simulink model "AeroPistonEngineSimulator"  (R2026a)
settings: Solver=VariableStepAuto  StopTime=1000
model workspace (MAT data in the model file):
  linear_friction_constant = 0.001
values from neighbouring files (symbols this model uses):
  C_oil = 2500    [engine_params.m]
  CHT_capacity = 100    [engine_params.m]
  drift_ialt = 0    [engine_params.m]
  drift_injd = 0    [engine_params.m]
  drift_injt = 0    [engine_params.m]
  drift_vbatt = 0    [engine_params.m]
  EGT_tau = 0.8    [engine_params.m]
  fault_ramp_time = 300    [engine_params.m]
  friction_a = 0.001    [engine_params.m]
  friction_b = 0.00005    (= 5e-05)    [engine_params.m]
  J_engine = 0.05    [engine_params.m]
  k_c = 5    [engine_params.m]
  k_h = 100    [engine_params.m]
  k_oil_cool = 0.05    [engine_params.m]
  k_oil_heat = 8    [engine_params.m]
  k_oil_pressure_rpm = 0.015    [engine_params.m]
  k_oil_pressure_temp = 0.000075    (= 7.5e-05)    [engine_params.m]
  RPM_max = 7500    [engine_params.m]
  sat_ialt = [0 40]    [engine_params.m]
  sat_injd = [0 30]    [engine_params.m]
  sat_injt = [0 60]    [engine_params.m]
  sat_vbatt = [0 36]    [engine_params.m]
  T_max = 10    [engine_params.m]
  tau_ialt_sensor = 0.1    [engine_params.m]
  tau_injd_sensor = 0.05    [engine_params.m]
  tau_injt_sensor = 0.05    [engine_params.m]
  tau_vbatt_sensor = 0.1    [engine_params.m]
  Ts_telemetry_slow = 0.5    [engine_params.m]
  Ts_telemetry_std = 0.1    [engine_params.m]
undefined symbols (not defined in the file or in its folder): DiscIntNeverNeededParam, elec, inj
libraries: simulink x27
settings Model: Creator=ambar  LastModifiedBy=vedanth
settings DataIOCC: LoadExternalInput=on

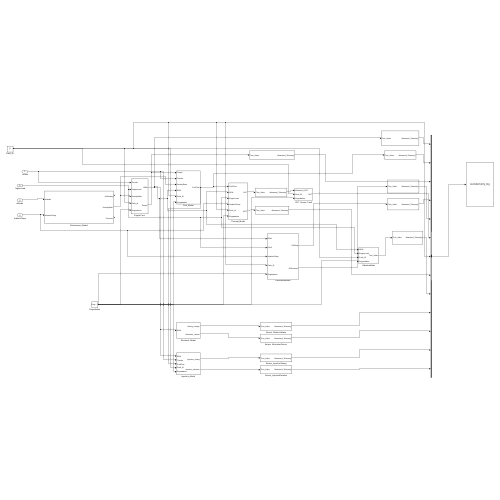
[thumbnail: Simulink's stored preview of the top-level diagram]
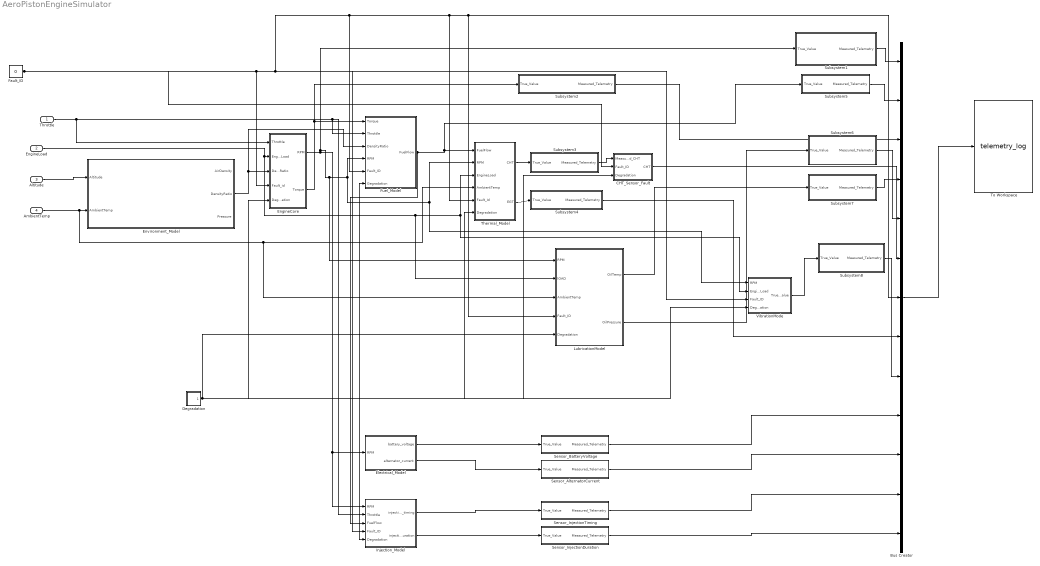
== system AeroPistonEngineSimulator ==
  Throttle : Inport
  EngineLoad : Inport  Port=2
  Altitude : Inport  Port=3
  AmbientTemp : Inport  Port=4
  Bus Creator : BusCreator  Inputs=13
  CHT_Sensor_Fault : Subsystem  Description=Fault 7 (CHT sensor drift/failure): the reported CHT drifts high and becomes erratic; the true engine CHT is unaffected. Pass-through for every other fault.
  Degradation : Subsystem  Description=Fault progression 0 -> 1. Starts at Fault_Onset (sim time the current fault was injected; set live by simulink_mqtt_stream.m) and rises at Progression_Rate per second. Fault tables clip at 1.
  Electrical_Model : Subsystem  Description=Read-only 28 VDC electrical system (parameters elec.* in engine_params.m). Input: engine RPM. Outputs: battery_voltage (V), alternator_current (A). No alternator torque is fed back into EngineCore.
  EngineCore : Subsystem
  Environment_Model : Subsystem
  Fault_ID : Constant  Value=0
  Fuel_Model : Subsystem
  Injection_Model : Subsystem  Description=|
      | Read-only ECU injection parameters (inj.* in engine_params.m). injection_timing = start of injection, deg BTDC, 2-D map of RPM x throttle. injection_duration = pulse width per event, ms, from fuel flow (kg/h) and RPM. Not fed back into combustion physics.
      | Fault 5 (injector abnormality): delivered fuel = k * commanded; the ECU pulse is computed from the full demand (measured fuel flow / k).
  LubricationModel : Subsystem
  Sensor_AlternatorCurrent : Subsystem
  Sensor_BatteryVoltage : Subsystem
  Sensor_InjectionDuration : Subsystem
  Sensor_InjectionTiming : Subsystem
  Subsystem1 : Subsystem
  Subsystem2 : Subsystem
  Subsystem3 : Subsystem
  Subsystem4 : Subsystem
  Subsystem5 : Subsystem
  Subsystem6 : Subsystem
  Subsystem7 : Subsystem
  Subsystem8 : Subsystem
  Thermal_Model : Subsystem
  To Workspace : ToWorkspace  VariableName=telemetry_log  SaveFormat=Timeseries  SampleTime=-1
  VibrationMode : Subsystem  Description=Fault 9 (abnormal vibration: imbalance / bearing wear): vibration amplitude grows with fault progression.
  wires:
  Bus Creator/1 -> To Workspace/1
  Throttle/1 -> Injection_Model/2(Throttle), Fuel_Model/2(Throttle), EngineCore/1(Throttle)
  Subsystem2/1(Measured_Telemetry) -> Bus Creator/3
  Fault_ID/1 -> Injection_Model/4(Fault_ID), Fuel_Model/5(Fault_ID), Thermal_Model/5(Fault_Id), Bus Creator/7, LubricationModel/4(Fault_ID), EngineCore/4(Fault_id), CHT_Sensor_Fault/2(Fault_ID), VibrationMode/3(Fault_ID)
  Fuel_Model/1(FuelFlow) -> Subsystem5/1(True_Value), Thermal_Model/1(FuelFlow), Injection_Model/3(FuelFlow)
  Altitude/1 -> Environment_Model/1(Altitude)
  EngineCore/1(RPM) -> Electrical_Model/1(RPM), Injection_Model/1(RPM), Subsystem1/1(True_Value), LubricationModel/1(RPM), VibrationMode/1(RPM), Thermal_Model/2(RPM), Fuel_Model/4(RPM)
  LubricationModel/2(OilPressure) -> Subsystem6/1(True_Value)
  Environment_Model/2(DensityRatio) -> Fuel_Model/3(DensityRatio), EngineCore/3(DensityRatio)
  EngineLoad/1 -> LubricationModel/2(lOAD), Thermal_Model/3(EngineLoad), VibrationMode/2(EngineLoad), EngineCore/2(EngineLoad)
  AmbientTemp/1 -> LubricationModel/3(AmbientTemp), Thermal_Model/4(AmbientTemp), Environment_Model/2(AmbientTemp)
  Subsystem7/1(Measured_Telemetry) -> Bus Creator/4
  VibrationMode/1(True_Value) -> Subsystem8/1(True_Value)
  Subsystem4/1(Measured_Telemetry) -> Bus Creator/8
  Subsystem6/1(Measured_Telemetry) -> Bus Creator/5
  Subsystem8/1(Measured_Telemetry) -> Bus Creator/9
  Subsystem1/1(Measured_Telemetry) -> Bus Creator/1
  EngineCore/2(Torque) -> Subsystem2/1(True_Value), Fuel_Model/1(Torque)
  Thermal_Model/2(EGT) -> Subsystem4/1(True_Value)
  Subsystem5/1(Measured_Telemetry) -> Bus Creator/2
  Thermal_Model/1(CHT) -> Subsystem3/1(True_Value)
  LubricationModel/1(OilTemp) -> Subsystem7/1(True_Value)
  Electrical_Model/1(battery_voltage) -> Sensor_BatteryVoltage/1(True_Value)
  Electrical_Model/2(alternator_current) -> Sensor_AlternatorCurrent/1(True_Value)
  Injection_Model/1(injection_timing) -> Sensor_InjectionTiming/1(True_Value)
  Injection_Model/2(injection_duration) -> Sensor_InjectionDuration/1(True_Value)
  Sensor_BatteryVoltage/1(Measured_Telemetry) -> Bus Creator/10
  Sensor_AlternatorCurrent/1(Measured_Telemetry) -> Bus Creator/11
  Sensor_InjectionTiming/1(Measured_Telemetry) -> Bus Creator/12
  Sensor_InjectionDuration/1(Measured_Telemetry) -> Bus Creator/13
  Degradation/1(Degradation) -> Injection_Model/5(Degradation), Fuel_Model/6(Gegradation), Thermal_Model/6(Degradation), LubricationModel/5(Degradation), EngineCore/5(Degradation), CHT_Sensor_Fault/3(Degradation), VibrationMode/4(Degradation)
  Subsystem3/1(Measured_Telemetry) -> CHT_Sensor_Fault/1(Measured_CHT)
  CHT_Sensor_Fault/1(CHT) -> Bus Creator/6

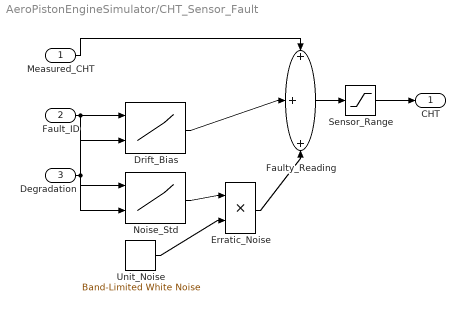
== system AeroPistonEngineSimulator/CHT_Sensor_Fault ==
  Measured_CHT : Inport
  Fault_ID : Inport  Port=2
  Degradation : Inport  Port=3
  Drift_Bias : Lookup_n-D  BreakpointsForDimension1=[0 1 2 3 4 5 6 7 8 9]  BreakpointsForDimension2=[0 0.25 0.5 0.75 1]  Table=[0 0 0 0 0;0 0 0 0 0;0 0 0 0 0;0 0 0 0 0;0 0 0 0 0;0 0 0 0 0;0 0 0 0 0;0 10 20 30 40;0 0 0 0 0;0 0 0 0 0]  ExtrapMethod=Clip  InternalRulePriority=Speed  RndMeth=Simplest
      settings: InputPortMap=u0,u1
  Erratic_Noise : Product
  Faulty_Reading : Sum  Inputs=+++
  Noise_Std : Lookup_n-D  BreakpointsForDimension1=[0 1 2 3 4 5 6 7 8 9]  BreakpointsForDimension2=[0 0.25 0.5 0.75 1]  Table=[0 0 0 0 0;0 0 0 0 0;0 0 0 0 0;0 0 0 0 0;0 0 0 0 0;0 0 0 0 0;0 0 0 0 0;0 1 2.5 4 6;0 0 0 0 0;0 0 0 0 0]  ExtrapMethod=Clip  InternalRulePriority=Speed  RndMeth=Simplest
      settings: InputPortMap=u0,u1
  Sensor_Range : Saturate  UpperLimit=300  LowerLimit=0
  Unit_Noise : simulink/Sources/Band-Limited White Noise  Cov=Ts_telemetry_slow  Ts=Ts_telemetry_slow  seed=23361
  CHT : Outport
  wires:
  Fault_ID/1 -> Drift_Bias/1, Noise_Std/1
  Degradation/1 -> Drift_Bias/2, Noise_Std/2
  Noise_Std/1 -> Erratic_Noise/1
  Unit_Noise/1 -> Erratic_Noise/2
  Measured_CHT/1 -> Faulty_Reading/1
  Drift_Bias/1 -> Faulty_Reading/2
  Erratic_Noise/1 -> Faulty_Reading/3
  Faulty_Reading/1 -> Sensor_Range/1
  Sensor_Range/1 -> CHT/1

== system AeroPistonEngineSimulator/Degradation ==
  Clock : Clock
  Fault_Onset : Constant  Value=0
  Not_Before_Onset : Saturate  UpperLimit=inf  LowerLimit=0
  Progression_Rate : Gain  Gain=1/fault_ramp_time
  Since_Onset : Sum  Inputs=+-
  Degradation : Outport
  wires:
  Clock/1 -> Since_Onset/1
  Fault_Onset/1 -> Since_Onset/2
  Since_Onset/1 -> Progression_Rate/1
  Progression_Rate/1 -> Not_Before_Onset/1
  Not_Before_Onset/1 -> Degradation/1

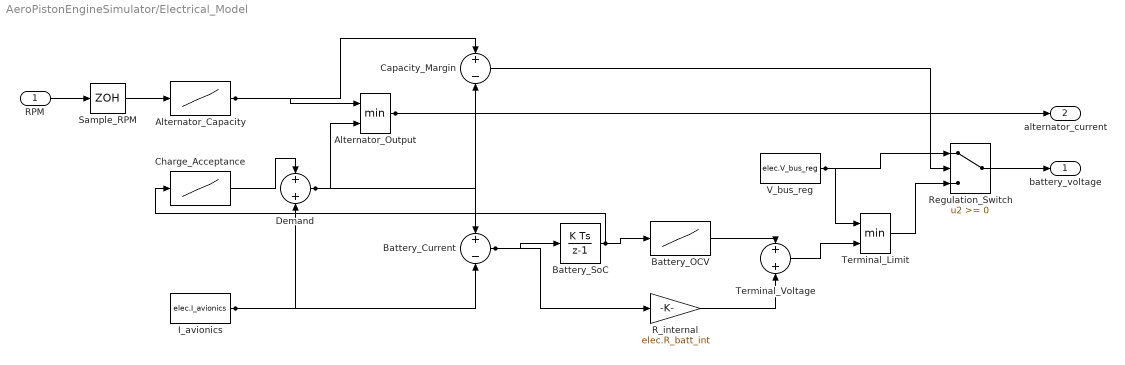
== system AeroPistonEngineSimulator/Electrical_Model ==
  RPM : Inport
  Alternator_Capacity : Lookup_n-D  NumberOfTableDimensions=1  BreakpointsForDimension1=[elec.RPM_alt_cutin elec.RPM_alt_rated]  Table=[0 elec.I_alt_max]  ExtrapMethod=Clip  InternalRulePriority=Speed  RndMeth=Simplest
  Alternator_Output : MinMax  Inputs=2  ZeroCross=off
  Battery_Current : Sum  Inputs=+-
  Battery_OCV : Lookup_n-D  NumberOfTableDimensions=1  BreakpointsForDimension1=[0 1]  Table=[elec.V_batt_empty elec.V_batt_full]  ExtrapMethod=Clip  InternalRulePriority=Speed  RndMeth=Simplest
  Battery_SoC : DiscreteIntegrator  gainval=1/(elec.C_batt_Ah*3600)  InitialCondition=elec.SoC_init  SampleTime=Ts_telemetry_std  LimitOutput=on  UpperSaturationLimit=1  LowerSaturationLimit=0  ICPrevOutput=DiscIntNeverNeededParam  ICPrevScaledInput=DiscIntNeverNeededParam
  Capacity_Margin : Sum  Inputs=+-
  Charge_Acceptance : Lookup_n-D  NumberOfTableDimensions=1  BreakpointsForDimension1=[elec.SoC_taper 1]  Table=[elec.I_charge_max 0]  ExtrapMethod=Clip  InternalRulePriority=Speed  RndMeth=Simplest
  Demand : Sum
  I_avionics : Constant  Value=elec.I_avionics  SampleTime=Ts_telemetry_std
  R_internal : Gain  Gain=elec.R_batt_int
  Regulation_Switch : Switch  ZeroCross=off  SaturateOnIntegerOverflow=off  InputSameDT=off
  Sample_RPM : ZeroOrderHold  SampleTime=Ts_telemetry_std
  Terminal_Limit : MinMax  Inputs=2  ZeroCross=off
  Terminal_Voltage : Sum
  V_bus_reg : Constant  Value=elec.V_bus_reg  SampleTime=Ts_telemetry_std
  battery_voltage : Outport
  alternator_current : Outport  Port=2
  wires:
  RPM/1 -> Sample_RPM/1
  Sample_RPM/1 -> Alternator_Capacity/1
  Battery_SoC/1 -> Charge_Acceptance/1, Battery_OCV/1
  Charge_Acceptance/1 -> Demand/1
  I_avionics/1 -> Demand/2, Battery_Current/2
  Alternator_Capacity/1 -> Alternator_Output/1, Capacity_Margin/1
  Demand/1 -> Alternator_Output/2, Capacity_Margin/2
  Alternator_Output/1 -> Battery_Current/1, alternator_current/1
  Battery_Current/1 -> Battery_SoC/1, R_internal/1
  Battery_OCV/1 -> Terminal_Voltage/1
  R_internal/1 -> Terminal_Voltage/2
  V_bus_reg/1 -> Terminal_Limit/1, Regulation_Switch/1
  Terminal_Voltage/1 -> Terminal_Limit/2
  Capacity_Margin/1 -> Regulation_Switch/2
  Terminal_Limit/1 -> Regulation_Switch/3
  Regulation_Switch/1 -> battery_voltage/1

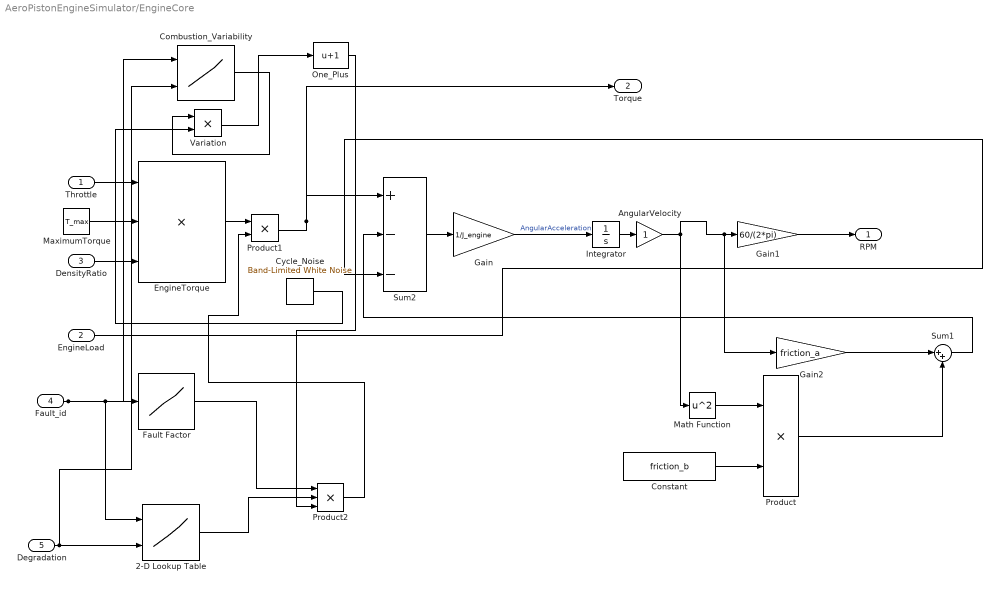
== system AeroPistonEngineSimulator/EngineCore ==
  Throttle : Inport
  EngineLoad : Inport  Port=2
  DensityRatio : Inport  Port=3
  Fault_id : Inport  Port=4
  Degradation : Inport  Port=5
  2-D Lookup Table : Lookup_n-D  BreakpointsForDimension1=[0 1 2 3 4 5 6 7 8 9]  BreakpointsForDimension2=[0 0.25 0.5 0.75 1]  Table=[1 1 1 1 1;1 0.9125 0.825 0.7375 0.65;1 1 1 1 1;1 1 1 1 1;1 0.8 0.6 0.4 0.2;1 0.96 0.92 0.88 0.84;1 1 1 1 1;1 1 1 1 1;1 0.99 0.98 0.97 0.96;1 0.995 0.99 0.985 0.98]  InterpMethod=Linear Lagrange  ExtrapMethod=Clip  InternalRulePriority=Speed  RndMeth=Simplest
      settings: InputPortMap=u0,u1
  AngularVelocity : Gain
  Combustion_Variability : Lookup_n-D  BreakpointsForDimension1=[0 1 2 3 4 5 6 7 8 9]  BreakpointsForDimension2=[0 0.25 0.5 0.75 1]  Table=[0 0 0 0 0;0 0 0 0 0;0 0 0 0 0;0 0 0 0 0;0 0 0 0 0;0 0 0 0 0;0 0 0 0 0;0 0 0 0 0;0 0.05 0.1 0.15 0.2;0 0 0 0 0]  ExtrapMethod=Clip  InternalRulePriority=Speed  RndMeth=Simplest
      settings: InputPortMap=u0,u1
  Constant : Constant  Value=friction_b
  Cycle_Noise : simulink/Sources/Band-Limited White Noise  Cov=0.05  Ts=0.05  seed=23381
  EngineTorque : Product  Inputs=3
  Fault Factor : Lookup_n-D  NumberOfTableDimensions=1  BreakpointsForDimension1=[0 1 2 3 4 5 6 7 8 9]  Table=[1 1 1 1 1 1 1 1 1 1]  InternalRulePriority=Speed  RndMeth=Simplest
  Gain : Gain  Gain=1/J_engine
  Gain1 : Gain  Gain=60/(2*pi)
  Gain2 : Gain  Gain=friction_a
  Integrator : Integrator
  Math Function : Math  Operator=square
  MaximumTorque : Constant  Value=T_max  VectorParams1D=off
  One_Plus : Bias  Bias=1  SaturateOnIntegerOverflow=off
  Product : Product
  Product1 : Product
  Product2 : Product  Inputs=3
  Sum1 : Sum  Inputs=|++
  Sum2 : Sum  Inputs=|+--
  Variation : Product
  RPM : Outport
  Torque : Outport  Port=2
  wires:
  Throttle/1 -> EngineTorque/1
  DensityRatio/1 -> EngineTorque/3
  MaximumTorque/1 -> EngineTorque/2
  EngineTorque/1 -> Product1/1
  EngineLoad/1 -> Sum2/3
  Sum2/1 -> Gain/1
  Gain/1 -> Integrator/1  "AngularAcceleration"
  Gain1/1 -> RPM/1
  Integrator/1 -> AngularVelocity/1
  AngularVelocity/1 -> Gain1/1, Gain2/1, Math Function/1
  Math Function/1 -> Product/1
  Constant/1 -> Product/2
  Gain2/1 -> Sum1/1
  Product/1 -> Sum1/2
  Sum1/1 -> Sum2/2
  Fault_id/1 -> 2-D Lookup Table/1, Fault Factor/1, Combustion_Variability/1
  Product1/1 -> Torque/1, Sum2/1
  2-D Lookup Table/1 -> Product2/2
  Fault Factor/1 -> Product2/1
  Product2/1 -> Product1/2
  Degradation/1 -> 2-D Lookup Table/2, Combustion_Variability/2
  Combustion_Variability/1 -> Variation/1
  Cycle_Noise/1 -> Variation/2
  Variation/1 -> One_Plus/1
  One_Plus/1 -> Product2/3

== system AeroPistonEngineSimulator/Environment_Model ==
  Altitude : Inport
  AmbientTemp : Inport  Port=2
  MATLAB Function : MATLAB Function  TreatAsAtomicUnit=on
  AirDensity : Outport
  DensityRatio : Outport  Port=2
  Pressure : Outport  Port=3
  wires:
  Altitude/1 -> MATLAB Function/1(altitude)
  AmbientTemp/1 -> MATLAB Function/2(temp_celsius)
  MATLAB Function/2(density) -> AirDensity/1
  MATLAB Function/3(density_ratio) -> DensityRatio/1
  MATLAB Function/1(pressure) -> Pressure/1

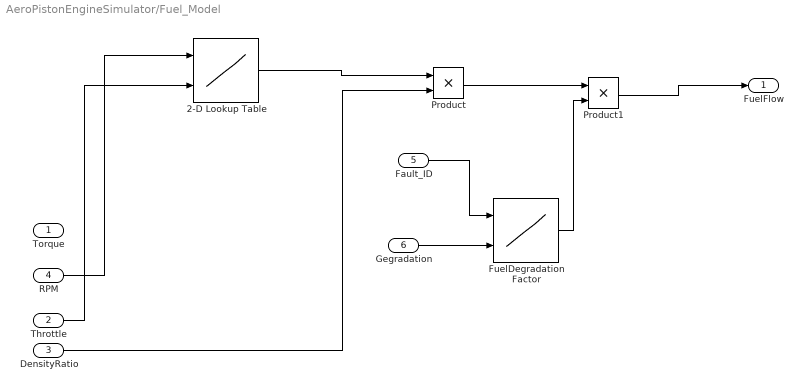
== system AeroPistonEngineSimulator/Fuel_Model ==
  Torque : Inport
  Throttle : Inport  Port=2
  DensityRatio : Inport  Port=3
  RPM : Inport  Port=4
  Fault_ID : Inport  Port=5
  Gegradation : Inport  Port=6
  2-D Lookup Table : Lookup_n-D  BreakpointsForDimension1=[1500, 3000, 5000, 7000]  BreakpointsForDimension2=[0.2, 0.5, 0.8, 1.0]  Table=[0.5 0.8 1.2 1.5; 1.0 1.5 2.0 2.5; 1.8 2.2 2.8 3.5; 2.5 3.0 3.8 4.5]  InternalRulePriority=Speed  RndMeth=Simplest
      settings: InputPortMap=u0,u1
  FuelDegradation Factor : Lookup_n-D  BreakpointsForDimension1=[0 1 2 3 4 5 6 7 8 9]  BreakpointsForDimension2=[0 0.25 0.5 0.75 1]  Table=[1 1 1 1 1;1 1 1 1 1;1 1 1 1 1;1 1 1 1 1;1 0.8 0.6 0.4 0.2;1 0.92 0.85 0.78 0.7;1 1 1 1 1;1 1 1 1 1;1 1 1 1 1;1 1 1 1 1]  InterpMethod=Linear Lagrange  ExtrapMethod=Clip  InternalRulePriority=Speed  RndMeth=Simplest
      settings: InputPortMap=u0,u1
  Product : Product
  Product1 : Product
  FuelFlow : Outport
  wires:
  RPM/1 -> 2-D Lookup Table/1
  Throttle/1 -> 2-D Lookup Table/2
  2-D Lookup Table/1 -> Product/1
  DensityRatio/1 -> Product/2
  Product/1 -> Product1/1
  Fault_ID/1 -> FuelDegradation Factor/1
  FuelDegradation Factor/1 -> Product1/2
  Product1/1 -> FuelFlow/1
  Gegradation/1 -> FuelDegradation Factor/2

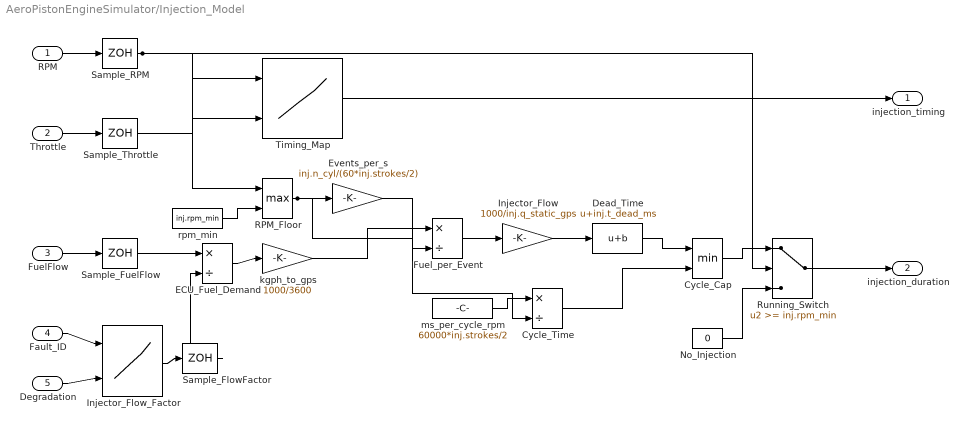
== system AeroPistonEngineSimulator/Injection_Model ==
  RPM : Inport
  Throttle : Inport  Port=2
  FuelFlow : Inport  Port=3
  Fault_ID : Inport  Port=4
  Degradation : Inport  Port=5
  Cycle_Cap : MinMax  Inputs=2  ZeroCross=off
  Cycle_Time : Product  Inputs=*/
  Dead_Time : Bias  Bias=inj.t_dead_ms  SaturateOnIntegerOverflow=off
  ECU_Fuel_Demand : Product  Inputs=*/
  Events_per_s : Gain  Gain=inj.n_cyl/(60*inj.strokes/2)
  Fuel_per_Event : Product  Inputs=*/
  Injector_Flow : Gain  Gain=1000/inj.q_static_gps
  Injector_Flow_Factor : Lookup_n-D  BreakpointsForDimension1=[0 1 2 3 4 5 6 7 8 9]  BreakpointsForDimension2=[0 0.25 0.5 0.75 1]  Table=[1 1 1 1 1;1 1 1 1 1;1 1 1 1 1;1 1 1 1 1;1 1 1 1 1;1 0.92 0.85 0.78 0.7;1 1 1 1 1;1 1 1 1 1;1 1 1 1 1;1 1 1 1 1]  ExtrapMethod=Clip  InternalRulePriority=Speed  RndMeth=Simplest
      settings: InputPortMap=u0,u1
  No_Injection : Constant  Value=0  SampleTime=Ts_telemetry_std
  RPM_Floor : MinMax  Function=max  Inputs=2  ZeroCross=off
  Running_Switch : Switch  Threshold=inj.rpm_min  ZeroCross=off  SaturateOnIntegerOverflow=off  InputSameDT=off
  Sample_FlowFactor : ZeroOrderHold  SampleTime=Ts_telemetry_std
  Sample_FuelFlow : ZeroOrderHold  SampleTime=Ts_telemetry_std
  Sample_RPM : ZeroOrderHold  SampleTime=Ts_telemetry_std
  Sample_Throttle : ZeroOrderHold  SampleTime=Ts_telemetry_std
  Timing_Map : Lookup_n-D  BreakpointsForDimension1=inj.rpm_bp  BreakpointsForDimension2=inj.throttle_bp  Table=inj.timing_table  ExtrapMethod=Clip  InternalRulePriority=Speed  RndMeth=Simplest
      settings: InputPortMap=u0,u1
  kgph_to_gps : Gain  Gain=1000/3600
  ms_per_cycle_rpm : Constant  Value=60000*inj.strokes/2  SampleTime=Ts_telemetry_std
  rpm_min : Constant  Value=inj.rpm_min  SampleTime=Ts_telemetry_std
  injection_timing : Outport
  injection_duration : Outport  Port=2
  wires:
  RPM/1 -> Sample_RPM/1
  Throttle/1 -> Sample_Throttle/1
  FuelFlow/1 -> Sample_FuelFlow/1
  Sample_RPM/1 -> Timing_Map/1, RPM_Floor/1, Running_Switch/2
  Sample_Throttle/1 -> Timing_Map/2
  Timing_Map/1 -> injection_timing/1
  rpm_min/1 -> RPM_Floor/2
  RPM_Floor/1 -> Events_per_s/1, Cycle_Time/2
  kgph_to_gps/1 -> Fuel_per_Event/1
  Events_per_s/1 -> Fuel_per_Event/2
  Fuel_per_Event/1 -> Injector_Flow/1
  Injector_Flow/1 -> Dead_Time/1
  ms_per_cycle_rpm/1 -> Cycle_Time/1
  Dead_Time/1 -> Cycle_Cap/1
  Cycle_Time/1 -> Cycle_Cap/2
  Cycle_Cap/1 -> Running_Switch/1
  No_Injection/1 -> Running_Switch/3
  Running_Switch/1 -> injection_duration/1
  Fault_ID/1 -> Injector_Flow_Factor/1
  Degradation/1 -> Injector_Flow_Factor/2
  Injector_Flow_Factor/1 -> Sample_FlowFactor/1
  Sample_FuelFlow/1 -> ECU_Fuel_Demand/1
  Sample_FlowFactor/1 -> ECU_Fuel_Demand/2
  ECU_Fuel_Demand/1 -> kgph_to_gps/1

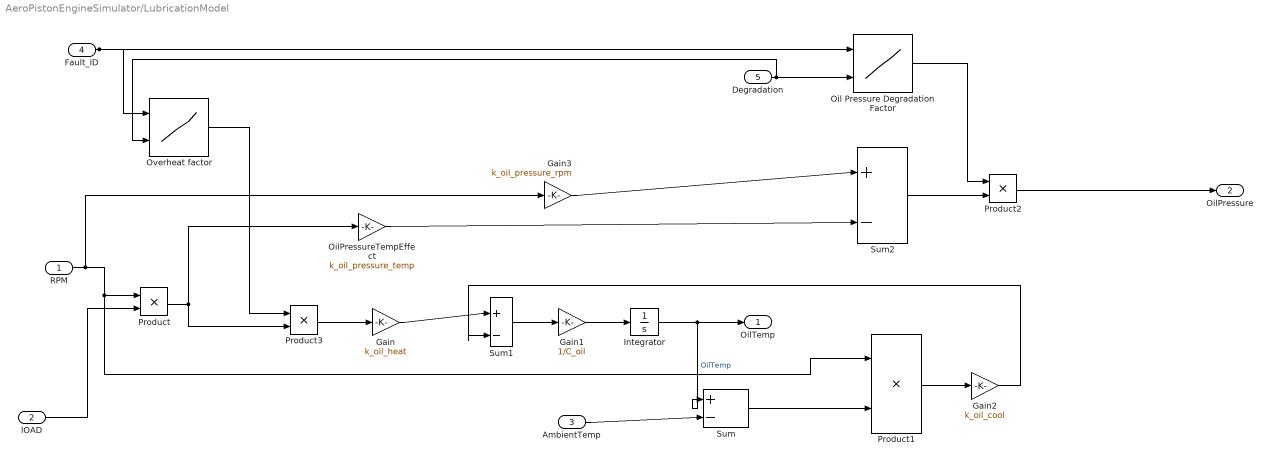
== system AeroPistonEngineSimulator/LubricationModel ==
  RPM : Inport
  lOAD : Inport  Port=2
  AmbientTemp : Inport  Port=3
  Fault_ID : Inport  Port=4
  Degradation : Inport  Port=5
  Gain : Gain  Gain=k_oil_heat
  Gain1 : Gain  Gain=1/C_oil
  Gain2 : Gain  Gain=k_oil_cool
  Gain3 : Gain  Gain=k_oil_pressure_rpm
  Integrator : Integrator  InitialCondition=25
  Oil Pressure Degradation Factor : Lookup_n-D  BreakpointsForDimension1=[0 1 2 3 4 5 6 7 8 9]  BreakpointsForDimension2=[0 0.25 0.5 0.75 1]  Table=[1 1 1 1 1;1 1 1 1 1;1 1 1 1 1;1 0.8 0.6 0.4 0.2;1 1 1 1 1;1 1 1 1 1;1 1 1 1 1;1 1 1 1 1;1 1 1 1 1;1 1 1 1 1]  InterpMethod=Linear Lagrange  ExtrapMethod=Clip  InternalRulePriority=Speed  RndMeth=Simplest
      settings: InputPortMap=u0,u1
  OilPressureTempEffect : Gain  Gain=k_oil_pressure_temp
  Overheat factor : Lookup_n-D  BreakpointsForDimension1=[0 1 2 3 4 5 6 7 8 9]  BreakpointsForDimension2=[0 0.25 0.5 0.75 1]  Table=[1 1 1 1 1;1 1 1 1 1;1 1.125 1.25 1.375 1.5;1 1.25 1.5 1.75 2;1 1.375 1.75 2.125 2.5;1 1 1 1 1;1 1.075 1.15 1.225 1.3;1 1 1 1 1;1 1 1 1 1;1 1 1 1 1]  ExtrapMethod=Clip  InternalRulePriority=Speed  RndMeth=Simplest
      settings: InputPortMap=u0,u1
  Product{,1..3} (4 alike) : Product
  Sum : Sum  Inputs=|+-
  Sum1 : Sum  Inputs=|+-
  Sum2 : Sum  Inputs=|+-
  OilTemp : Outport
  OilPressure : Outport  Port=2
  wires:
  RPM/1 -> Gain3/1, Product1/1, Product/1
  lOAD/1 -> Product/2
  Product/1 -> Product3/2, OilPressureTempEffect/1
  AmbientTemp/1 -> Sum/2
  Gain/1 -> Sum1/1
  Sum1/1 -> Gain1/1
  Gain1/1 -> Integrator/1
  Integrator/1 -> Sum/1, OilTemp/1  "OilTemp"
  Sum/1 -> Product1/2
  Product1/1 -> Gain2/1
  Gain2/1 -> Sum1/2
  Gain3/1 -> Sum2/1
  Product2/1 -> OilPressure/1
  OilPressureTempEffect/1 -> Sum2/2
  Sum2/1 -> Product2/2
  Fault_ID/1 -> Oil Pressure Degradation Factor/1, Overheat factor/1
  Oil Pressure Degradation Factor/1 -> Product2/1
  Degradation/1 -> Oil Pressure Degradation Factor/2, Overheat factor/2
  Product3/1 -> Gain/1
  Overheat factor/1 -> Product3/1

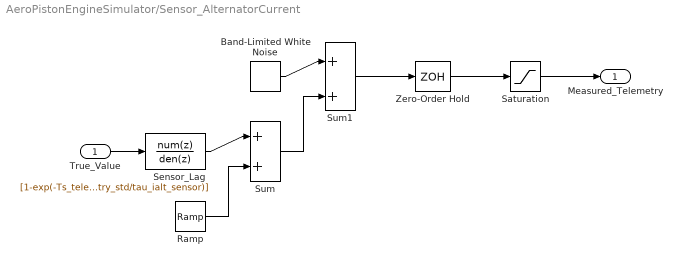
== system AeroPistonEngineSimulator/Sensor_AlternatorCurrent ==
  True_Value : Inport
  Band-Limited White Noise : simulink/Sources/Band-Limited White Noise  Cov=noise_ialt  Ts=Ts_telemetry_std  seed=seed_ialt
  Ramp : simulink/Sources/Ramp  slope=drift_ialt  start=0  InitialOutput=0
  Saturation : Saturate  UpperLimit=sat_ialt(2)  LowerLimit=sat_ialt(1)
  Sensor_Lag : DiscreteTransferFcn  Numerator=[1-exp(-Ts_telemetry_std/tau_ialt_sensor)]  Denominator=[1 -exp(-Ts_telemetry_std/tau_ialt_sensor)]  SampleTime=Ts_telemetry_std
  Sum : Sum  Inputs=|++
  Sum1 : Sum  Inputs=|++
  Zero-Order Hold : ZeroOrderHold  SampleTime=Ts_telemetry_std
  Measured_Telemetry : Outport
  wires:
  Saturation/1 -> Measured_Telemetry/1
  Zero-Order Hold/1 -> Saturation/1
  Sum1/1 -> Zero-Order Hold/1
  Sum/1 -> Sum1/2
  Band-Limited White Noise/1 -> Sum1/1
  Ramp/1 -> Sum/2
  True_Value/1 -> Sensor_Lag/1
  Sensor_Lag/1 -> Sum/1

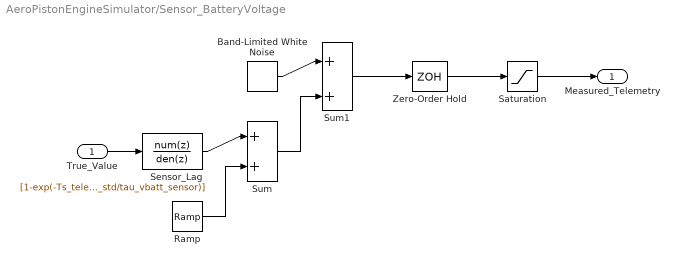
== system AeroPistonEngineSimulator/Sensor_BatteryVoltage ==
  True_Value : Inport
  Band-Limited White Noise : simulink/Sources/Band-Limited White Noise  Cov=noise_vbatt  Ts=Ts_telemetry_std  seed=seed_vbatt
  Ramp : simulink/Sources/Ramp  slope=drift_vbatt  start=0  InitialOutput=0
  Saturation : Saturate  UpperLimit=sat_vbatt(2)  LowerLimit=sat_vbatt(1)
  Sensor_Lag : DiscreteTransferFcn  Numerator=[1-exp(-Ts_telemetry_std/tau_vbatt_sensor)]  Denominator=[1 -exp(-Ts_telemetry_std/tau_vbatt_sensor)]  SampleTime=Ts_telemetry_std
  Sum : Sum  Inputs=|++
  Sum1 : Sum  Inputs=|++
  Zero-Order Hold : ZeroOrderHold  SampleTime=Ts_telemetry_std
  Measured_Telemetry : Outport
  wires:
  Saturation/1 -> Measured_Telemetry/1
  Zero-Order Hold/1 -> Saturation/1
  Sum1/1 -> Zero-Order Hold/1
  Sum/1 -> Sum1/2
  Band-Limited White Noise/1 -> Sum1/1
  Ramp/1 -> Sum/2
  True_Value/1 -> Sensor_Lag/1
  Sensor_Lag/1 -> Sum/1

== system AeroPistonEngineSimulator/Sensor_InjectionDuration ==
  True_Value : Inport
  Band-Limited White Noise : simulink/Sources/Band-Limited White Noise  Cov=noise_injd  Ts=Ts_telemetry_std  seed=seed_injd
  Ramp : simulink/Sources/Ramp  slope=drift_injd  start=0  InitialOutput=0
  Saturation : Saturate  UpperLimit=sat_injd(2)  LowerLimit=sat_injd(1)
  Sensor_Lag : DiscreteTransferFcn  Numerator=[1-exp(-Ts_telemetry_std/tau_injd_sensor)]  Denominator=[1 -exp(-Ts_telemetry_std/tau_injd_sensor)]  SampleTime=Ts_telemetry_std
  Sum : Sum  Inputs=|++
  Sum1 : Sum  Inputs=|++
  Zero-Order Hold : ZeroOrderHold  SampleTime=Ts_telemetry_std
  Measured_Telemetry : Outport
  wires:
  Saturation/1 -> Measured_Telemetry/1
  Zero-Order Hold/1 -> Saturation/1
  Sum1/1 -> Zero-Order Hold/1
  Sum/1 -> Sum1/2
  Band-Limited White Noise/1 -> Sum1/1
  Ramp/1 -> Sum/2
  True_Value/1 -> Sensor_Lag/1
  Sensor_Lag/1 -> Sum/1

== system AeroPistonEngineSimulator/Sensor_InjectionTiming ==
  True_Value : Inport
  Band-Limited White Noise : simulink/Sources/Band-Limited White Noise  Cov=noise_injt  Ts=Ts_telemetry_std  seed=seed_injt
  Ramp : simulink/Sources/Ramp  slope=drift_injt  start=0  InitialOutput=0
  Saturation : Saturate  UpperLimit=sat_injt(2)  LowerLimit=sat_injt(1)
  Sensor_Lag : DiscreteTransferFcn  Numerator=[1-exp(-Ts_telemetry_std/tau_injt_sensor)]  Denominator=[1 -exp(-Ts_telemetry_std/tau_injt_sensor)]  SampleTime=Ts_telemetry_std
  Sum : Sum  Inputs=|++
  Sum1 : Sum  Inputs=|++
  Zero-Order Hold : ZeroOrderHold  SampleTime=Ts_telemetry_std
  Measured_Telemetry : Outport
  wires:
  Saturation/1 -> Measured_Telemetry/1
  Zero-Order Hold/1 -> Saturation/1
  Sum1/1 -> Zero-Order Hold/1
  Sum/1 -> Sum1/2
  Band-Limited White Noise/1 -> Sum1/1
  Ramp/1 -> Sum/2
  True_Value/1 -> Sensor_Lag/1
  Sensor_Lag/1 -> Sum/1

== system AeroPistonEngineSimulator/Subsystem1 ==
  True_Value : Inport
  Band-Limited White Noise : simulink/Sources/Band-Limited White Noise  Cov=[0.01]  Ts=0.1  seed=[23341]
  Ramp : simulink/Sources/Ramp  slope=0  start=0  InitialOutput=0
  Saturation : Saturate  UpperLimit=9000  LowerLimit=0
  Sum : Sum  Inputs=|++
  Sum1 : Sum  Inputs=|++
  Transfer Fcn : TransferFcn  Denominator=[0.05 1]
  Zero-Order Hold : ZeroOrderHold  SampleTime=0.05
  Measured_Telemetry : Outport
  wires:
  True_Value/1 -> Transfer Fcn/1
  Transfer Fcn/1 -> Sum/1
  Ramp/1 -> Sum/2
  Band-Limited White Noise/1 -> Sum1/1
  Sum/1 -> Sum1/2
  Sum1/1 -> Zero-Order Hold/1
  Zero-Order Hold/1 -> Saturation/1
  Saturation/1 -> Measured_Telemetry/1

== system AeroPistonEngineSimulator/Subsystem2 ==
  True_Value : Inport
  Band-Limited White Noise : simulink/Sources/Band-Limited White Noise  Cov=[0.1]  Ts=0.1  seed=[23341]
  Ramp : simulink/Sources/Ramp  slope=0.001  start=0  InitialOutput=0
  Saturation : Saturate  UpperLimit=10  LowerLimit=-10
  Sum : Sum  Inputs=|++
  Sum1 : Sum  Inputs=|++
  Transfer Fcn : TransferFcn  Denominator=[1 1]
  Zero-Order Hold : ZeroOrderHold  SampleTime=-1
  Measured_Telemetry : Outport
  wires:
  True_Value/1 -> Transfer Fcn/1
  Transfer Fcn/1 -> Sum/1
  Ramp/1 -> Sum/2
  Band-Limited White Noise/1 -> Sum1/1
  Sum/1 -> Sum1/2
  Sum1/1 -> Zero-Order Hold/1
  Zero-Order Hold/1 -> Saturation/1
  Saturation/1 -> Measured_Telemetry/1

== system AeroPistonEngineSimulator/Subsystem3 ==
  True_Value : Inport
  Band-Limited White Noise : simulink/Sources/Band-Limited White Noise  Cov=0.05  Ts=0.1  seed=[23341]
  Ramp : simulink/Sources/Ramp  slope=0.001  start=0  InitialOutput=0
  Saturation : Saturate  UpperLimit=300  LowerLimit=0
  Sum : Sum  Inputs=|++
  Sum1 : Sum  Inputs=|++
  Transfer Fcn : TransferFcn  Denominator=[3 1]
  Zero-Order Hold : ZeroOrderHold  SampleTime=0.5
  Measured_Telemetry : Outport
  wires:
  True_Value/1 -> Transfer Fcn/1
  Transfer Fcn/1 -> Sum/1
  Ramp/1 -> Sum/2
  Band-Limited White Noise/1 -> Sum1/1
  Sum/1 -> Sum1/2
  Sum1/1 -> Zero-Order Hold/1
  Zero-Order Hold/1 -> Saturation/1
  Saturation/1 -> Measured_Telemetry/1

== system AeroPistonEngineSimulator/Subsystem4 ==
  True_Value : Inport
  Band-Limited White Noise : simulink/Sources/Band-Limited White Noise  Cov=[0.2]  Ts=0.1  seed=[23341]
  Ramp : simulink/Sources/Ramp  slope=0  start=0  InitialOutput=0
  Saturation : Saturate  UpperLimit=1500  LowerLimit=0
  Sum : Sum  Inputs=|++
  Sum1 : Sum  Inputs=|++
  Transfer Fcn : TransferFcn  Denominator=[0.8 1]
  Zero-Order Hold : ZeroOrderHold  SampleTime=0.1
  Measured_Telemetry : Outport
  wires:
  True_Value/1 -> Transfer Fcn/1
  Transfer Fcn/1 -> Sum/1
  Ramp/1 -> Sum/2
  Band-Limited White Noise/1 -> Sum1/1
  Sum/1 -> Sum1/2
  Sum1/1 -> Zero-Order Hold/1
  Zero-Order Hold/1 -> Saturation/1
  Saturation/1 -> Measured_Telemetry/1

== system AeroPistonEngineSimulator/Subsystem5 ==
  True_Value : Inport
  Band-Limited White Noise : simulink/Sources/Band-Limited White Noise  Cov=[0.001]  Ts=0.1  seed=[23341]
  Ramp : simulink/Sources/Ramp  slope=0  start=0  InitialOutput=0
  Saturation : Saturate  UpperLimit=10  LowerLimit=0
  Sum : Sum  Inputs=|++
  Sum1 : Sum  Inputs=|++
  Transfer Fcn : TransferFcn  Denominator=[0.2 1]
  Zero-Order Hold : ZeroOrderHold  SampleTime=0.2
  Measured_Telemetry : Outport
  wires:
  True_Value/1 -> Transfer Fcn/1
  Transfer Fcn/1 -> Sum/1
  Ramp/1 -> Sum/2
  Band-Limited White Noise/1 -> Sum1/1
  Sum/1 -> Sum1/2
  Sum1/1 -> Zero-Order Hold/1
  Zero-Order Hold/1 -> Saturation/1
  Saturation/1 -> Measured_Telemetry/1

== system AeroPistonEngineSimulator/Subsystem6 ==
  True_Value : Inport
  Band-Limited White Noise : simulink/Sources/Band-Limited White Noise  Cov=0.05  Ts=0.1  seed=[23341]
  Ramp : simulink/Sources/Ramp  slope=-0.0005  start=0  InitialOutput=0
  Saturation : Saturate  UpperLimit=150  LowerLimit=0
  Sum : Sum  Inputs=|++
  Sum1 : Sum  Inputs=|++
  Transfer Fcn : TransferFcn  Denominator=[0.1 1]
  Zero-Order Hold : ZeroOrderHold  SampleTime=0.1
  Measured_Telemetry : Outport
  wires:
  True_Value/1 -> Transfer Fcn/1
  Transfer Fcn/1 -> Sum/1
  Ramp/1 -> Sum/2
  Band-Limited White Noise/1 -> Sum1/1
  Sum/1 -> Sum1/2
  Sum1/1 -> Zero-Order Hold/1
  Zero-Order Hold/1 -> Saturation/1
  Saturation/1 -> Measured_Telemetry/1

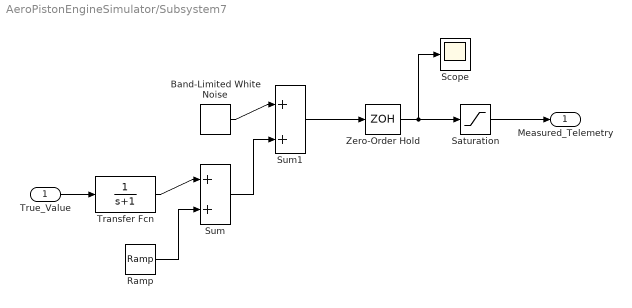
== system AeroPistonEngineSimulator/Subsystem7 ==
  True_Value : Inport
  Band-Limited White Noise : simulink/Sources/Band-Limited White Noise  Cov=[0.1]  Ts=0.1  seed=[23341]
  Ramp : simulink/Sources/Ramp  slope=0.001  start=0  InitialOutput=0
  Saturation : Saturate  UpperLimit=150  LowerLimit=0
  Scope : Scope
      settings: ActiveDisplayYMinimum=-75.19425986782052  ActiveDisplayYMaximum=450.06365181654218  DataLoggingVariableName=ScopeData3
  Sum : Sum  Inputs=|++
  Sum1 : Sum  Inputs=|++
  Transfer Fcn : TransferFcn  Denominator=[1 1]
  Zero-Order Hold : ZeroOrderHold  SampleTime=-1
  Measured_Telemetry : Outport
  wires:
  True_Value/1 -> Transfer Fcn/1
  Transfer Fcn/1 -> Sum/1
  Ramp/1 -> Sum/2
  Band-Limited White Noise/1 -> Sum1/1
  Sum/1 -> Sum1/2
  Sum1/1 -> Zero-Order Hold/1
  Zero-Order Hold/1 -> Scope/1, Saturation/1
  Saturation/1 -> Measured_Telemetry/1

== system AeroPistonEngineSimulator/Subsystem8 ==
  True_Value : Inport
  Band-Limited White Noise : simulink/Sources/Band-Limited White Noise  Cov=[0.1]  Ts=0.1  seed=[23341]
  Ramp : simulink/Sources/Ramp  slope=0  start=0  InitialOutput=0
  Saturation : Saturate  UpperLimit=20  LowerLimit=-20
  Sum : Sum  Inputs=|++
  Sum1 : Sum  Inputs=|++
  Transfer Fcn : TransferFcn  Denominator=[0.005 1]
  Zero-Order Hold : ZeroOrderHold  SampleTime=0.005
  Measured_Telemetry : Outport
  wires:
  True_Value/1 -> Transfer Fcn/1
  Transfer Fcn/1 -> Sum/1
  Ramp/1 -> Sum/2
  Band-Limited White Noise/1 -> Sum1/1
  Sum/1 -> Sum1/2
  Sum1/1 -> Zero-Order Hold/1
  Zero-Order Hold/1 -> Saturation/1
  Saturation/1 -> Measured_Telemetry/1

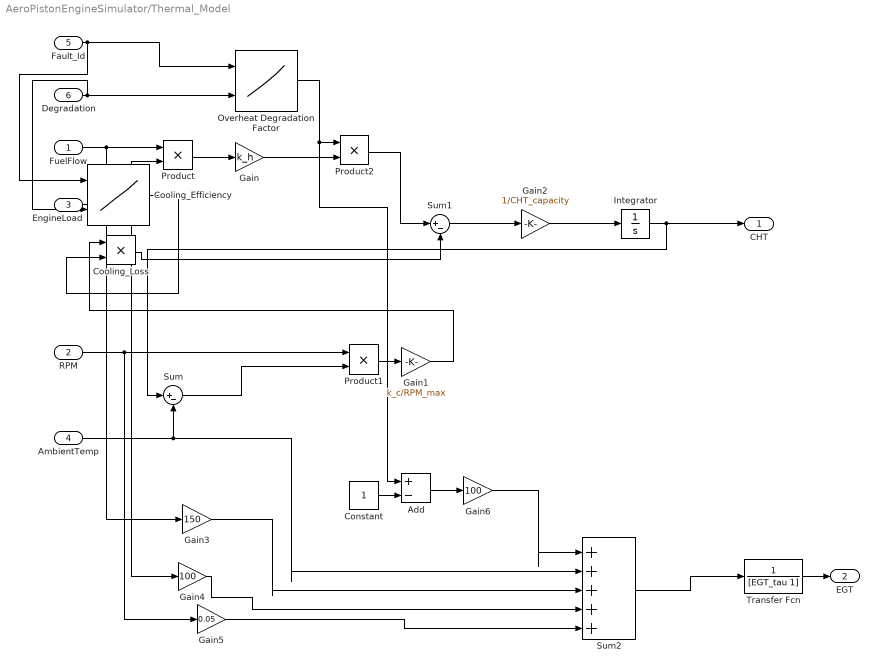
== system AeroPistonEngineSimulator/Thermal_Model ==
  FuelFlow : Inport
  RPM : Inport  Port=2
  EngineLoad : Inport  Port=3
  AmbientTemp : Inport  Port=4
  Fault_Id : Inport  Port=5
  Degradation : Inport  Port=6
  Add : Sum  Inputs=+-
  Constant : Constant
  Cooling_Efficiency : Lookup_n-D  BreakpointsForDimension1=[0 1 2 3 4 5 6 7 8 9]  BreakpointsForDimension2=[0 0.25 0.5 0.75 1]  Table=[1 1 1 1 1;1 1 1 1 1;1 1 1 1 1;1 1 1 1 1;1 1 1 1 1;1 1 1 1 1;1 0.85 0.7 0.55 0.4;1 1 1 1 1;1 1 1 1 1;1 1 1 1 1]  ExtrapMethod=Clip  InternalRulePriority=Speed  RndMeth=Simplest
      settings: InputPortMap=u0,u1
  Cooling_Loss : Product
  Gain : Gain  Gain=k_h
  Gain1 : Gain  Gain=k_c/RPM_max
  Gain2 : Gain  Gain=1/CHT_capacity
  Gain3 : Gain  Gain=150
  Gain4 : Gain  Gain=100
  Gain5 : Gain  Gain=0.05
  Gain6 : Gain  Gain=100
  Integrator : Integrator  InitialCondition=25
  Overheat Degradation Factor : Lookup_n-D  BreakpointsForDimension1=[0 1 2 3 4 5 6 7 8 9]  BreakpointsForDimension2=[0 0.25 0.5 0.75 1]  Table=[1 1 1 1 1;1 1 1 1 1;1 1.75 2.5 3.25 4;1 1 1 1 1;1 1 1 1 1;1 1 1 1 1;1 1 1 1 1;1 1 1 1 1;1 1 1 1 1;1 1 1 1 1]  InterpMethod=Linear Lagrange  ExtrapMethod=Clip  InternalRulePriority=Speed  RndMeth=Simplest
      settings: InputPortMap=u0,u1
  Product : Product
  Product1 : Product
  Product2 : Product
  Sum : Sum  Inputs=|+-
  Sum1 : Sum  Inputs=|+-
  Sum2 : Sum  Inputs=|+++++
  Transfer Fcn : TransferFcn  Denominator=[EGT_tau 1]
  CHT : Outport
  EGT : Outport  Port=2
  wires:
  FuelFlow/1 -> Product/1, Gain3/1
  EngineLoad/1 -> Gain4/1, Product/2
  Product/1 -> Gain/1
  AmbientTemp/1 -> Sum2/2, Sum/2
  RPM/1 -> Gain5/1, Product1/1
  Sum/1 -> Product1/2
  Product1/1 -> Gain1/1
  Sum1/1 -> Gain2/1
  Integrator/1 -> CHT/1, Sum/1
  Gain2/1 -> Integrator/1
  Gain5/1 -> Sum2/5
  Sum2/1 -> Transfer Fcn/1
  Transfer Fcn/1 -> EGT/1
  Fault_Id/1 -> Overheat Degradation Factor/1, Cooling_Efficiency/1
  Product2/1 -> Sum1/1
  Degradation/1 -> Overheat Degradation Factor/2, Cooling_Efficiency/2
  Gain/1 -> Product2/2
  Gain4/1 -> Sum2/4
  Overheat Degradation Factor/1 -> Product2/1, Add/1
  Gain3/1 -> Sum2/3
  Constant/1 -> Add/2
  Add/1 -> Gain6/1
  Gain6/1 -> Sum2/1
  Gain1/1 -> Cooling_Loss/1
  Cooling_Efficiency/1 -> Cooling_Loss/2
  Cooling_Loss/1 -> Sum1/2

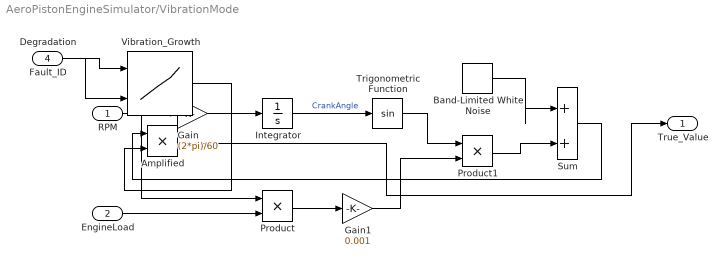
== system AeroPistonEngineSimulator/VibrationMode ==
  RPM : Inport
  EngineLoad : Inport  Port=2
  Fault_ID : Inport  Port=3
  Degradation : Inport  Port=4
  Amplified : Product
  Band-Limited White Noise : simulink/Sources/Band-Limited White Noise  Cov=[0.1]  Ts=0.1  seed=[23341]
  Gain : Gain  Gain=(2*pi)/60
  Gain1 : Gain  Gain=0.001
  Integrator : Integrator
  Product : Product
  Product1 : Product
  Sum : Sum  Inputs=|++
  Trigonometric Function : Trigonometry
  Vibration_Growth : Lookup_n-D  BreakpointsForDimension1=[0 1 2 3 4 5 6 7 8 9]  BreakpointsForDimension2=[0 0.25 0.5 0.75 1]  Table=[1 1 1 1 1;1 1 1 1 1;1 1 1 1 1;1 1 1 1 1;1 1 1 1 1;1 1 1 1 1;1 1 1 1 1;1 1 1 1 1;1 1 1 1 1;1 1.6 2.3 3.1 4]  ExtrapMethod=Clip  InternalRulePriority=Speed  RndMeth=Simplest
      settings: InputPortMap=u0,u1
  True_Value : Outport
  wires:
  RPM/1 -> Product/1, Gain/1
  Gain/1 -> Integrator/1
  Integrator/1 -> Trigonometric Function/1  "CrankAngle"
  EngineLoad/1 -> Product/2
  Product/1 -> Gain1/1
  Trigonometric Function/1 -> Product1/1
  Gain1/1 -> Product1/2
  Product1/1 -> Sum/2
  Band-Limited White Noise/1 -> Sum/1
  Sum/1 -> Amplified/1
  Vibration_Growth/1 -> Amplified/2
  Amplified/1 -> True_Value/1
  Fault_ID/1 -> Vibration_Growth/1
  Degradation/1 -> Vibration_Growth/2

== matlab function AeroPistonEngineSimulator/Environment_Model/MATLAB Function ==
  data: altitude input; pressure output; temp_celsius input; density output; density_ratio output
function [pressure, density, density_ratio] = calculate_atmosphere(altitude, temp_celsius)
    % Standard ISA Constants
    P0 = 101325;       % Sea level standard pressure (Pa)
    T0 = 288.15;       % Sea level standard temperature (K)
    rho0 = 1.225;      % Sea level standard density (kg/m^3)
    L = 0.0065;        % Temperature lapse rate (K/m)
    R = 287.05;        % Specific gas constant for dry air (J/(kg*K))
    g = 9.80665;       % Gravity (m/s^2)
    
    % Convert input temp to Kelvin
    T_ambient = temp_celsius + 273.15;
    
    % Calculate pressure at altitude
    % Assuming troposphere (under ~11,000m)
    pressure = P0 * (1 - (L * altitude) / T0) ^ ((g) / (R * L));
    
    % Calculate current air density (Ideal Gas Law: P = rho * R * T)
    density = pressure / (R * T_ambient);
    
    % Calculate density ratio (sigma)
    density_ratio = density / rho0;
end
